simulink model "Simulink_Model"  (R2023a)
settings: Solver=VariableStepAuto  StartTime=0.0  StopTime=0.15  RelTol=1e-3
model workspace (MAT data in the model file):
  y = 0.001
undefined symbols (not defined in the file or in its folder): D1, Delta, x
libraries: spsCurrentMeasurementLib x4, spsDistributedParametersLineLib x3, spsThreePhaseVIMeasurementLib x2, spsThreePhaseParallelRLCLoadLib x1, spsThreePhaseTransformerTwoWindingsLib x1, spsThreePhaseFaultLib x1, spsThreePhaseSourceLib x1, spsVoltageMeasurementLib x1, spspowerguiLib x1
settings Model: Creator=Krish Sanjay Shah  LastModifiedBy=Krish Sanjay Shah

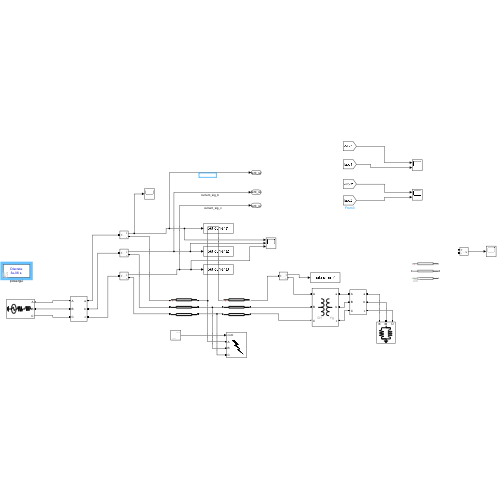
[thumbnail: Simulink's stored preview of the top-level diagram]
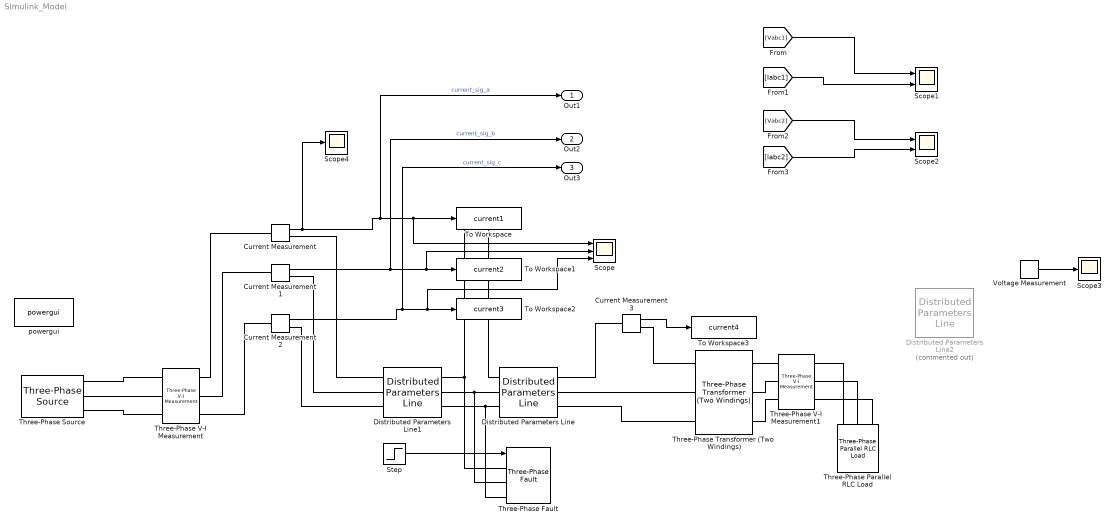
== system Simulink_Model ==
  Current Measurement{,1..3} (4 alike) : spsCurrentMeasurementLib/Current Measurement  PhasorSimulation=off  OutputType=Complex  PSBequivalent=0
  Distributed Parameters Line : spsDistributedParametersLineLib/Distributed Parameters Line  Phases=3  Length=100-x  Frequency=50  Resistance=[0.01273 0.3864]  Inductance="[0.9337e-3  4.1264e-3]"  Capacitance=[12.74e-9 7.751e-9]  x1=[-0.000555 -5.58295531136589e-12 3727.3774424138 -10318.9689781437;-0.000552 -5.5777870589433e-12 3737.10118466611 -10315.4514252007;-0.000549 -5.57261385197143e-12 3746.82160738473 -10311.9247094101;-0.000546 -5.56743569504544e-12 3756.53870193537 -10308.3888339046;-0.000543 -5.56225259276491e-12 3766.25245968668 -10304.8438018251;-0.00054 -5.55706454973381e-12 3775.96287201026 -10301.2896163203;-0.000537 -5.55187157056049e-12 3785.66993028072 -10297.7262805474;-0.000534 -5.54667365985768e-12 3795.3736258756 -10294.1537976716;-0.000531 -5.54147082224252e-12 3805.07395017548 -10290.5721708661;-0.000528 -5.53626306233648e-12 3814.77089456389 -10286.9814033125;-0.000525 -5.53105038476544e-12 3824.46445042739 -10283.3814982002;-0.000522 -5.52583279415963e-12 3834.15460915553 -10279.7724587269;-0.000519 -5.52061029515366e-12 3843.84136214089 -10276.1542880984;-0.000516 -5.51538289238648e-12 3853.52470077909 -10272.5269895286;-0.000513 -5.51015059050141e-12 3863.20461646874 -10268.8905662395;-0.00051 -5.50491339414612e-12 3872.88110061154 -10265.2450214612;-0.000507 -5.49967130797261e-12 3882.55414461219 -10261.5903584319;-0.000504 -5.49442433663725e-12 3892.22373987849 -10257.9265803979;-0.000501 -5.48917248480074e-12 3901.88987782128 -10254.2536906137;-0.000498 -5.48391575712811e-12 3911.55254985446 -10250.5716923416;-0.000495 -5.47865415828872e-12 3921.21174739504 -10246.8805888524;-0.000492 -5.47338769295627e-12 3930.86746186309 -10243.1803834246;-0.000489 -5.46811636580876e-12 3940.51968468179 -10239.471079345;-0.000486 -5.46284018152852e-12 3950.16840727741 -10235.7526799086;-0.000483 -5.45755914480222e-12 3959.81362107934 -10232.0251884181;-0.00048 -5.45227326032079e-12 3969.45531752007 -10228.2886081846;-0.000477 -5.44698253277951e-12 3979.09348803523 -10224.5429425272;-0.000474 -5.44168696687793e-12 3988.72812406358 -10220.7881947731;-0.000471 -5.43638656731993e-12 3998.35921704701 -10217.0243682573;-0.000468 -5.43108133881365e-12 4007.98675843057 -10213.2514663232;-0.000465 -5.42577128607154e-12 4017.61073966246 -10209.4694923222;-0.000462 -5.42045641381034e-12 4027.23115219403 -10205.6784496135;-0.000459 -5.41513672675104e-12 4036.84798747982 -10201.8783415648;-0.000456 -5.40981222961895e-12 4046.46123697754 -10198.0691715514;-0.000453 -5.40448292714363e-12 4056.07089214807 -10194.2509429569;-0.00045 -5.39914882405889e-12 4065.67694445551 -10190.4236591729;-0.000447 -5.39380992510284e-12 4075.27938536714 -10186.5873235991;-0.000444 -5.38846623501783e-12 4084.87820635346 -10182.7419396431;-0.000441 -5.38311775855047e-12 4094.47339888817 -10178.8875107207;-0.000438 -5.37776450045161e-12 4104.06495444821 -10175.0240402555;-0.000435 -5.37240646547637e-12 4113.65286451374 -10171.1515316795;-0.000432 -5.3670436583841e-12 4123.23712056817 -10167.2699884323;-0.000429 -5.3616760839384e-12 4132.81771409814 -10163.3794139619;-0.000426 -5.35630374690707e-12 4142.39463659354 -10159.4798117241;-0.000423 -5.35092665206218e-12 4151.96787954755 -10155.5711851827;-0.00042 -5.34554480418002e-12 4161.53743445659 -10151.6535378097;-0.000417 -5.34015820804108e-12 4171.10329282037 -10147.726873085;-0.000414 -5.33476686843008e-12 4180.66544614187 -10143.7911944964;-0.000411 -5.32937079013596e-12 4190.22388592739 -10139.84650554;-0.000408 -5.32396997795187e-12 4199.77860368648 -10135.8928097196;-0.000405 -5.31856443667515e-12 4209.32959093205 -10131.9301105471;-0.000402 -5.31315417110735e-12 4218.87683918029 -10127.9584115426;-0.000399 -5.30773918605422e-12 4228.42033995072 -10123.9777162338;-0.000396 -5.3023194863257e-12 4237.96008476619 -10119.9880281568;-0.000393 -5.29689507673591e-12 4247.49606515288 -10115.9893508554;-0.00039 -5.29146596210316e-12 4257.02827264032 -10111.9816878814;-0.000387 -5.28603214724994e-12 4266.55669876139 -10107.9650427948;-0.000384 -5.28059363700292e-12 4276.08133505234 -10103.9394191635;-0.000381 -5.27515043619292e-12 4285.60217305276 -10099.9048205631;-0.000378 -5.26970254965496e-12 4295.11920430563 ...(+8296 chars)]  x2=[-0.000555 -8.16324412980977e-12 3109.62540123163 -10027.2164900334;-0.000552 -8.15415122200079e-12 3119.0744476462 -10024.2812841631;-0.000549 -8.14505107115012e-12 3128.52072349819 -10021.3371740814;-0.000546 -8.13594368534112e-12 3137.96422039683 -10018.3841624033;-0.000543 -8.12682907266356e-12 3147.40492995377 -10015.4222517518;-0.00054 -8.1177072412136e-12 3156.84284378318 -10012.4514447581;-0.000537 -8.10857819909387e-12 3166.27795350169 -10009.4717440608;-0.000534 -8.09944195441335e-12 3175.71025072844 -10006.4831523069;-0.000531 -8.09029851528744e-12 3185.13972708505 -10003.4856721509;-0.000528 -8.08114788983794e-12 3194.56637419566 -10000.4793062553;-0.000525 -8.07199008619302e-12 3203.9901836869 -9997.46405729078;-0.000522 -8.06282511248724e-12 3213.41114718795 -9994.43992793549;-0.000519 -8.0536529768615e-12 3222.8292563305 -9991.40692087572;-0.000516 -8.0444736874631e-12 3232.24450274877 -9988.36503880557;-0.000513 -8.03528725244566e-12 3241.65687807955 -9985.31428442703;-0.00051 -8.02609367996917e-12 3251.06637396215 -9982.25466044999;-0.000507 -8.01689297819996e-12 3260.47298203845 -9979.1861695922;-0.000504 -8.00768515531067e-12 3269.87669395291 -9976.10881457929;-0.000501 -7.99847021948029e-12 3279.27750135253 -9973.02259814476;-0.000498 -7.98924817889412e-12 3288.67539588692 -9969.92752302999;-0.000495 -7.98001904174376e-12 3298.07036920826 -9966.82359198423;-0.000492 -7.97078281622713e-12 3307.46241297134 -9963.71080776459;-0.000489 -7.96153951054844e-12 3316.85151883353 -9960.58917313603;-0.000486 -7.95228913291819e-12 3326.23767845482 -9957.4586908714;-0.000483 -7.94303169155316e-12 3335.62088349783 -9954.3193637514;-0.00048 -7.9337671946764e-12 3345.00112562779 -9951.17119456458;-0.000477 -7.92449565051724e-12 3354.37839651257 -9948.01418610733;-0.000474 -7.91521706731126e-12 3363.75268782267 -9944.84834118393;-0.000471 -7.90593145330029e-12 3373.12399123123 -9941.67366260648;-0.000468 -7.89663881673241e-12 3382.49229841408 -9938.49015319493;-0.000465 -7.88733916586194e-12 3391.85760104966 -9935.29781577707;-0.000462 -7.87803250894942e-12 3401.21989081913 -9932.09665318856;-0.000459 -7.86871885426164e-12 3410.57915940629 -9928.88666827286;-0.000456 -7.85939821007157e-12 3419.93539849763 -9925.66786388129;-0.000453 -7.85007058465841e-12 3429.28859978235 -9922.44024287301;-0.00045 -7.84073598630757e-12 3438.63875495233 -9919.20380811499;-0.000447 -7.83139442331062e-12 3447.98585570215 -9915.95856248204;-0.000444 -7.82204590396535e-12 3457.32989372913 -9912.7045088568;-0.000441 -7.81269043657571e-12 3466.67086073329 -9909.44165012973;-0.000438 -7.80332802945184e-12 3476.00874841737 -9906.1699891991;-0.000435 -7.79395869091001e-12 3485.34354848687 -9902.88952897102;-0.000432 -7.7845824292727e-12 3494.67525265002 -9899.60027235941;-0.000429 -7.77519925286848e-12 3504.0038526178 -9896.30222228599;-0.000426 -7.7658091700321e-12 3513.32934010394 -9892.9953816803;-0.000423 -7.75641218910444e-12 3522.65170682494 -9889.6797534797;-0.00042 -7.7470083184325e-12 3531.97094450009 -9886.35534062933;-0.000417 -7.73759756636941e-12 3541.28704485143 -9883.02214608216;-0.000414 -7.7281799412744e-12 3550.59999960381 -9879.68017279894;-0.000411 -7.7187554515128e-12 3559.90980048485 -9876.32942374822;-0.000408 -7.70932410545607e-12 3569.216439225 -9872.96990190637;-0.000405 -7.69988591148172e-12 3578.5199075575 -9869.60161025751;-0.000402 -7.69044087797336e-12 3587.82019721841 -9866.22455179359;-0.000399 -7.68098901332069e-12 3597.11729994662 -9862.83872951433;-0.000396 -7.67153032591946e-12 3606.41120748383 -9859.44414642722;-0.000393 -7.66206482417148e-12 3615.70191157461 -9856.04080554756;-0.00039 -7.65259251648462e-12 3624.98940396635 -9852.62870989842;-0.000387 -7.64311341127279e-12 3634.27367640931 -9849.20786251064;-0.000384 -7.63362751695595e-12 3643.5547206566 -9845.77826642283;-0.000381 -7.62413484196007e-12 3652.83252846418 -9842.33992468137;-0.000378 -7.61463539471716e-12 3662.10709159093 -9838.89284034044 ...(+8275 chars)]  x3=[-0.000555 -5.59033495049164e-14 20.8975033204712 -16.8365307190214;-0.000552 -5.59192310651593e-14 20.9133620932343 -16.8168278114194;-0.000549 -5.59350629543439e-14 20.9292022894038 -16.7971099660291;-0.000546 -5.59508451584073e-14 20.9450238949094 -16.7773772003651;-0.000543 -5.59665776633306e-14 20.9608268956974 -16.7576295319554;-0.00054 -5.59822604551393e-14 20.9766112777306 -16.7378669783411;-0.000537 -5.59978935199029e-14 20.9923770269882 -16.7180895570767;-0.000534 -5.60134768437352e-14 21.008124129466 -16.6982972857296;-0.000531 -5.60290104127939e-14 21.0238525711766 -16.6784901818806;-0.000528 -5.60444942132812e-14 21.0395623381488 -16.6586682631238;-0.000525 -5.60599282314434e-14 21.0552534164283 -16.6388315470661;-0.000522 -5.6075312453571e-14 21.0709257920772 -16.6189800513279;-0.000519 -5.60906468659987e-14 21.0865794511743 -16.5991137935424;-0.000516 -5.61059314551056e-14 21.102214379815 -16.5792327913563;-0.000513 -5.61211662073148e-14 21.1178305641114 -16.5593370624291;-0.00051 -5.61363511090939e-14 21.1334279901922 -16.5394266244334;-0.000507 -5.61514861469547e-14 21.1490066442027 -16.519501495055;-0.000504 -5.61665713074532e-14 21.164566512305 -16.4995616919927;-0.000501 -5.61816065771899e-14 21.1801075806778 -16.4796072329582;-0.000498 -5.61965919428094e-14 21.1956298355166 -16.4596381356765;-0.000495 -5.62115273910008e-14 21.2111332630333 -16.4396544178853;-0.000492 -5.62264129084975e-14 21.226617849457 -16.4196560973355;-0.000489 -5.62412484820772e-14 21.2420835810333 -16.3996431917909;-0.000486 -5.62560340985619e-14 21.2575304440243 -16.3796157190282;-0.000483 -5.62707697448182e-14 21.2729584247093 -16.3595736968371;-0.00048 -5.62854554077569e-14 21.2883675093842 -16.3395171430202;-0.000477 -5.63000910743333e-14 21.3037576843615 -16.3194460753931;-0.000474 -5.63146767315469e-14 21.3191289359708 -16.2993605117842;-0.000471 -5.63292123664419e-14 21.3344812505583 -16.2792604700347;-0.000468 -5.63436979661069e-14 21.3498146144871 -16.2591459679988;-0.000465 -5.63581335176747e-14 21.3651290141371 -16.2390170235434;-0.000462 -5.63725190083227e-14 21.3804244359051 -16.2188736545485;-0.000459 -5.63868544252729e-14 21.3957008662047 -16.1987158789067;-0.000456 -5.64011397557916e-14 21.4109582914664 -16.1785437145233;-0.000453 -5.64153749871897e-14 21.4261966981376 -16.1583571793167;-0.00045 -5.64295601068225e-14 21.4414160726825 -16.1381562912177;-0.000447 -5.64436951020899e-14 21.4566164015823 -16.1179410681702;-0.000444 -5.64577799604362e-14 21.4717976713351 -16.0977115281305;-0.000441 -5.64718146693505e-14 21.4869598684559 -16.0774676890678;-0.000438 -5.64857992163661e-14 21.5021029794768 -16.0572095689641;-0.000435 -5.6499733589061e-14 21.5172269909465 -16.0369371858139;-0.000432 -5.6513617775058e-14 21.532331889431 -16.0166505576244;-0.000429 -5.65274517620241e-14 21.5474176615131 -15.9963497024155;-0.000426 -5.65412355376711e-14 21.5624842937927 -15.9760346382198;-0.000423 -5.65549690897554e-14 21.5775317728866 -15.9557053830824;-0.00042 -5.6568652406078e-14 21.5925600854288 -15.935361955061;-0.000417 -5.65822854744844e-14 21.60756921807 -15.915004372226;-0.000414 -5.65958682828649e-14 21.6225591574782 -15.8946326526603;-0.000411 -5.66094008191544e-14 21.6375298903383 -15.8742468144593;-0.000408 -5.66228830713323e-14 21.6524814033525 -15.8538468757312;-0.000405 -5.66363150274229e-14 21.6674136832398 -15.8334328545963;-0.000402 -5.66496966754951e-14 21.6823267167363 -15.8130047691879;-0.000399 -5.66630280036624e-14 21.6972204905955 -15.7925626376513;-0.000396 -5.66763090000831e-14 21.7120949915876 -15.7721064781447;-0.000393 -5.66895396529601e-14 21.7269502065002 -15.7516363088384;-0.00039 -5.67027199505412e-14 21.7417861221379 -15.7311521479155;-0.000387 -5.67158498811187e-14 21.7566027253226 -15.7106540135713;-0.000384 -5.67289294330297e-14 21.771400002893 -15.6901419240135;-0.000381 -5.67419585946563e-14 21.7861779417055 -15.6696158974622;-0.000378 -5.67549373544249e-14 21.8009365286332 -15.6490759521502 ...(+8276 chars)]  x4=[-0.000555 -6.06778096436729e-15 0.285467066139237 -59.3990605496309;-0.000552 -6.07292661894897e-15 0.34144922674214 -59.398765122266;-0.000549 -6.07806687916656e-15 0.397431084047879 -59.3984169330968;-0.000546 -6.08320174045415e-15 0.453412588329759 -59.3980159824326;-0.000543 -6.08833119825061e-15 0.509393689861408 -59.3975622706294;-0.00054 -6.09345524799964e-15 0.565374338916814 -59.3970557980904;-0.000537 -6.09857388514973e-15 0.621354485770363 -59.3964965652654;-0.000534 -6.10368710515416e-15 0.677334080696882 -59.3958845726511;-0.000531 -6.10879490347106e-15 0.733313073971702 -59.3952198207912;-0.000528 -6.11389727556334e-15 0.789291415870672 -59.3945023102762;-0.000525 -6.11899421689875e-15 0.845269056670229 -59.3937320417433;-0.000522 -6.12408572294987e-15 0.90124594664744 -59.3929090158768;-0.000519 -6.12917178919407e-15 0.957222036080019 -59.3920332334078;-0.000516 -6.13425241111361e-15 1.01319727524641 -59.3911046951141;-0.000513 -6.13932758419553e-15 1.0691716144258 -59.3901234018206;-0.00051 -6.14439730393175e-15 1.12514500389818 -59.3890893543989;-0.000507 -6.14946156581901e-15 1.18111739394439 -59.3880025537675;-0.000504 -6.15452036535892e-15 1.23708873484615 -59.3868630008918;-0.000501 -6.15957369805791e-15 1.29305897688611 -59.385670696784;-0.000498 -6.16462155942729e-15 1.3490280703479 -59.3844256425031;-0.000495 -6.16966394498324e-15 1.40499596551618 -59.3831278391552;-0.000492 -6.17470085024677e-15 1.46096261267666 -59.381777287893;-0.000489 -6.17973227074378e-15 1.51692796211616 -59.3803739899162;-0.000486 -6.18475820200505e-15 1.57289196412266 -59.3789179464713;-0.000483 -6.18977863956622e-15 1.62885456898534 -59.3774091588515;-0.00048 -6.1947935789678e-15 1.6848157269946 -59.3758476283972;-0.000477 -6.19980301575522e-15 1.74077538844215 -59.3742333564953;-0.000474 -6.20480694547877e-15 1.79673350362101 -59.3725663445799;-0.000471 -6.20980536369362e-15 1.85269002282559 -59.3708465941315;-0.000468 -6.21479826595988e-15 1.90864489635171 -59.3690741066778;-0.000465 -6.21978564784251e-15 1.96459807449665 -59.3672488837933;-0.000462 -6.22476750491141e-15 2.02054950755919 -59.3653709270992;-0.000459 -6.22974383274137e-15 2.07649914583968 -59.3634402382636;-0.000456 -6.2347146269121e-15 2.13244693964005 -59.3614568190016;-0.000453 -6.23967988300821e-15 2.18839283926386 -59.3594206710749;-0.00045 -6.24463959661926e-15 2.24433679501637 -59.3573317962921;-0.000447 -6.24959376333969e-15 2.30027875720457 -59.3551901965087;-0.000444 -6.2545423787689e-15 2.35621867613719 -59.3529958736271;-0.000441 -6.25948543851122e-15 2.41215650212481 -59.3507488295963;-0.000438 -6.26442293817589e-15 2.46809218547985 -59.3484490664124;-0.000435 -6.26935487337712e-15 2.52402567651663 -59.3460965861181;-0.000432 -6.27428123973404e-15 2.57995692555144 -59.343691390803;-0.000429 -6.27920203287073e-15 2.63588588290254 -59.3412334826037;-0.000426 -6.28411724841624e-15 2.69181249889023 -59.3387228637033;-0.000423 -6.28902688200455e-15 2.74773672383689 -59.336159536332;-0.00042 -6.2939309292746e-15 2.80365850806703 -59.3335435027667;-0.000417 -6.29882938587031e-15 2.85957780190733 -59.3308747653312;-0.000414 -6.30372224744056e-15 2.91549455568666 -59.3281533263958;-0.000411 -6.30860950963919e-15 2.97140871973617 -59.3253791883781;-0.000408 -6.31349116812501e-15 3.02732024438931 -59.3225523537422;-0.000405 -6.31836721856183e-15 3.08322907998186 -59.319672824999;-0.000402 -6.32323765661842e-15 3.13913517685199 -59.3167406047064;-0.000399 -6.32810247796856e-15 3.19503848534032 -59.3137556954689;-0.000396 -6.33296167829098e-15 3.25093895578993 -59.3107180999379;-0.000393 -6.33781525326943e-15 3.30683653854642 -59.3076278208116;-0.00039 -6.34266319859267e-15 3.36273118395797 -59.304484860835;-0.000387 -6.34750550995442e-15 3.41862284237536 -59.3012892227999;-0.000384 -6.35234218305345e-15 3.47451146415201 -59.2980409095448;-0.000381 -6.3571732135935e-15 3.53039699964407 -59.2947399239551;-0.000378 -6.36199859728334e-15 3.5862793992104 ...(+8297 chars)]  x5=0.000554230735655828  V1=[9.004e-12 1.096e+04 1.096e+04;314.2 314.2 314.2;2.187 0.4167 -1.154]  V2=[2.274e-12 1.05e+04 1.05e+04;314.2 314.2 314.2;0.7585 0.3721 -1.199]  I1=[8.942e-14 26.84 26.84;314.2 314.2 314.2;-2.539 0.9674 -0.6034]  I2=[4.925e-14 59.41 59.41;314.2 314.2 314.2;1.818 0.07624 -1.495]  nHarmo=1  Measurements=None  Decoupling=off  VsMag0=0  VrMag0=0  VsAngle0=0  VrAngle0=0  IsMag0=0  IrMag0=0  IsAngle0=0  IrAngle0=0
      settings: LibrarySourceBlock=sps_lib/Power Grid Elements/Distributed Parameters Line
  Distributed Parameters Line1 : spsDistributedParametersLineLib/Distributed Parameters Line  Phases=3  Length=x  Frequency=50  Resistance=[0.01273 0.3864]  Inductance="[0.9337e-3  4.1264e-3]"  Capacitance=[12.74e-9 7.751e-9]  x1=[-1.2e-05 -1.83954871437303e-12 0 0;-9e-06 -1.83441132626429e-12 5446.91147624279 -9533.87651759339;-6e-06 -1.8292723087134e-12 5455.89452269233 -9528.73869092862;-3e-06 -1.82413166628518e-12 5464.87272286537 -9523.59240022514]  x2=[-1.2e-05 -4.57144213691916e-12 0 0;-9e-06 -4.56545605758146e-12 5434.03223661431 -9531.30405671462;-6e-06 -4.55946592291199e-12 5443.01286429704 -9526.17836958794;-3e-06 -4.55347173823158e-12 5451.98865714558 -9521.04422069681]  x3=[-1.2e-05 -1.5803084134562e-12 0 0;-9e-06 -1.57981970240911e-12 23.5061505546778 -13.1350607237431;-6e-06 -1.57932958806454e-12 23.5185196160898 -13.1129008683509;-3e-06 -1.57883807085782e-12 23.5308677868397 -13.0907293652366]  x4=[-1.2e-05 -5.34003166758131e-13 0 0;-9e-06 -5.32771603259301e-13 16.6074504479067 -57.3277256214439;-6e-06 -5.3153956651846e-13 16.6614731725027 -57.3120480093776;-3e-06 -5.30307057629981e-13 16.7154810973064 -57.2963194890633]  x5=1.13108313399149e-05  V1=[2.274e-12 1.098e+04 1.098e+04;314.2 314.2 314.2;0.9184 0.5165 -1.054]  V2=[9.004e-12 1.096e+04 1.096e+04;314.2 314.2 314.2;2.347 0.5142 -1.057]  I1=[1.903e-12 26.92 26.92;314.2 314.2 314.2;1.493 1.059 -0.5121]  I2=[1.719e-12 59.68 59.68;314.2 314.2 314.2;-0.7165 0.2761 -1.295]  nHarmo=1  Measurements=None  Decoupling=off  VsMag0=0  VrMag0=0  VsAngle0=0  VrAngle0=0  IsMag0=0  IrMag0=0  IsAngle0=0  IrAngle0=0
      settings: LibrarySourceBlock=sps_lib/Power Grid Elements/Distributed Parameters Line
  Distributed Parameters Line2 : spsDistributedParametersLineLib/Distributed Parameters Line  Commented=on  Phases=3  Length=100  Frequency=60  Resistance=[0.01273 0.3864]  Inductance="[0.9337e-3  4.1264e-3]"  Capacitance=[12.74e-9 7.751e-9]  x1=[0 0 0 0; 0.0001244 0 0 0; 0.0002488 0 0 0; 0.0003733 0 0 0; 0.0004977 0 0 0; 0.0006221 0 0 0]  x2=[0 0 0 0; 0.0001244 0 0 0; 0.0002488 0 0 0; 0.0003733 0 0 0; 0.0004977 0 0 0; 0.0006221 0 0 0]  x3=[0 0 0 0; 0.0001244 0 0 0; 0.0002488 0 0 0; 0.0003733 0 0 0; 0.0004977 0 0 0; 0.0006221 0 0 0]  x4=[0 0 0 0; 0.0001244 0 0 0; 0.0002488 0 0 0; 0.0003733 0 0 0; 0.0004977 0 0 0; 0.0006221 0 0 0]  x5=0  V1=ones(3,3)  V2=ones(3,3)  I1=ones(3,3)  I2=ones(3,3)  nHarmo=1  Measurements=None  Decoupling=off  VsMag0=0  VrMag0=0  VsAngle0=0  VrAngle0=0  IsMag0=0  IrMag0=0  IsAngle0=0  IrAngle0=0
      settings: LibrarySourceBlock=sps_lib/Power Grid Elements/Distributed Parameters Line
  Scope : Scope  NumInputPorts=3
  Scope1 : Scope  NumInputPorts=2
  Scope2 : Scope  NumInputPorts=2
  Scope3 : Scope
  Scope4 : Scope
  Step : Step  Time=t  SampleTime=0
  Three-Phase Parallel RLC Load : spsThreePhaseParallelRLCLoadLib/Three-Phase Parallel RLC Load  LConnTagsString=A|B|C  Configuration=Y (grounded)  NominalVoltage=0.4e3  Vabc=[1e3 1e3 1e3]  Vabcp=[1e3 1e3 1e3]  NominalFrequency=50  UnbalancedPower=off  ActivePower=10e3  InductivePower=100  CapacitivePower=0  Pabc=[10e3 9e3 11e3]  QLabc=[100 90 110]  QCabc=[100 90 110]  Pabcp=[10e3 9e3 11e3]  QLabcp=[100 90 110]  QCabcp=[100 90 110]  Measurements=None  LoadType=constant Z
  Three-Phase Transformer (Two Windings) : spsThreePhaseTransformerTwoWindingsLib/Three-Phase Transformer (Two Windings)  Winding1Connection=Delta (D1)  Winding2Connection=Yg  CoreType=Three single-phase transformers  SetSaturation=off  Hysteresis=off  DataFile='hysteresis'  SetInitialFlux=off  Measurements=None  UNITS=pu  NominalPower=[ 100e6 , 50 ]  Winding1=[ 11e3 , 0.002 , 0.08 ]  Winding2=[ 0.4e3 , 0.002 , 0.08 ]  Rm=500  Lm=500  L0=0.5  Saturation=[ 0,0 ; 0.0024,1.2 ; 1.0,1.52 ]  InitialFluxes=[ 0.8 , -0.8 , 0.7 ]  BreakLoop=off  DiscreteSolver=Trapezoidal iterative  DataType=off  TransfoNumber=1
  Three-Phase V-I Measurement : spsThreePhaseVIMeasurementLib/Three-Phase V-I Measurement  VoltageMeasurement=phase-to-ground  SetLabelV=on  LabelV=Vabc1  Vpu=off  VpuLL=off  CurrentMeasurement=yes  SetLabelI=on  LabelI=Iabc1  Ipu=off  Pbase=100e6  Vbase=500e3  OutputType=Complex  PhasorSimulation=off  PSBequivalent=0
  Three-Phase V-I Measurement1 : spsThreePhaseVIMeasurementLib/Three-Phase V-I Measurement  VoltageMeasurement=phase-to-ground  SetLabelV=on  LabelV=Vabc2  Vpu=off  VpuLL=off  CurrentMeasurement=yes  SetLabelI=on  LabelI=Iabc2  Ipu=off  Pbase=100e6  Vbase=500e3  OutputType=Complex  PhasorSimulation=off  PSBequivalent=0
  Three-Phase Fault : spsThreePhaseFaultLib/Three-Phase Fault  InitialStates=0  FaultA=on  FaultB=off  FaultC=off  GroundFault=on  SwitchTimes=0.05  External=on  SwitchStatus=NaN  FaultResistance=y  GroundResistance=0.01  SnubberResistance=1e6  SnubberCapacitance=inf  Measurements=None
  Three-Phase Source : spsThreePhaseSourceLib/Three-Phase Source  InternalConnection=Yg  VoltagePhases=off  Voltage=11e3  PhaseAngle=0  Voltage_phases=[25e3 25e3 25e3]/sqrt(3)  PhaseAngles_phases=[0 -120 +120]  Frequency=50  NonIdealSource=on  SpecifyImpedance=on  Resistance=0.8929  Inductance=16.58e-3  ShortCircuitLevel=100e6  BaseVoltage=11e3  XRratio=7  BusType=swing  Pref=10e3  Qref=0  Prefabc=[10e3, 10e3, 10e3]  Qrefabc=[0, 0, 0]  Qmin=-inf  Qmax=inf
  To Workspace : ToWorkspace  VariableName=current1  SaveFormat=Structure With Time  SampleTime=-1
  To Workspace1 : ToWorkspace  VariableName=current2  SaveFormat=Structure With Time  SampleTime=-1
  To Workspace2 : ToWorkspace  VariableName=current3  SaveFormat=Structure With Time  SampleTime=-1
  To Workspace3 : ToWorkspace  VariableName=current4  SaveFormat=Structure With Time  SampleTime=-1
  Voltage Measurement : spsVoltageMeasurementLib/Voltage Measurement  PhasorSimulation=off  OutputType=Complex  PSBequivalent=0
  powergui : spspowerguiLib/powergui  Priority=1  SimulationMode=Discrete  SampleTime=3e-06  frequency=60  Iterations=50  frequencyindice=50  Pbase=100e6  ErrMax=1e-4  UnitsV=kV  UnitsW=MW  buscounter=0  FunctionMessages=off  echomessages=off  EnableUseOfTLC=off  CurrentSourceSwitches=on  DisableSnubberDevices=off  DisableRonSwitches=off  DisableVfSwitches=off  DisplayEquations=off  AutomaticDiscreteSolvers=off  SolverType=Tustin/Backward Euler (TBE)  Interpol=off  ExternalGateDelay=off  methode=off  Ts=100  x0status=blocks  SPID=on  SwTol=0  HookPort=off  NonlinearTolerance=1e-4  nMaxIteration=100  ContinueOnMaxIteration=off  RestoreLinks=warning  ResistiveCurrentMeasurement=off  Frange=[0:2:500]  Ylog=off  Xlog=on  ShowGrid=off  save=off  variable=ZData  structure=0  ZoomFFT=off  StartTime=0.0  cycles=1  DisplayStyle=1  fundamental=60  FreqAxis=off  MaxFrequency=1000  frequencyindicesteady=1  RmsSteady=1  display=off
  Out1 : Outport
  Out2 : Outport  Port=2
  Out3 : Outport  Port=3
  wires:
  Current Measurement/1 -> Scope4/1, Out1/1, Scope/1, To Workspace/1  "current_sig_a"
  Current Measurement1/1 -> Out2/1, Scope/2, To Workspace1/1  "current_sig_b"
  Current Measurement2/1 -> Out3/1, Scope/3, To Workspace2/1  "current_sig_c"
  Current Measurement3/1 -> To Workspace3/1
  [Iabc2] -> Scope2/2
  [Iabc1] -> Scope1/2
  [Vabc2] -> Scope2/1
  [Vabc1] -> Scope1/1
  Voltage Measurement/1 -> Scope3/1
  Step/1 -> Three-Phase Fault/1
  connections:
  Three-Phase Source/RConn2 -- Three-Phase V-I Measurement/LConn2
  Three-Phase Source/RConn3 -- Three-Phase V-I Measurement/LConn3
  Three-Phase Source/RConn1 -- Three-Phase V-I Measurement/LConn1
  Three-Phase V-I Measurement/RConn3 -- Current Measurement2/LConn1
  Three-Phase V-I Measurement/RConn2 -- Current Measurement1/LConn1
  Three-Phase V-I Measurement/RConn1 -- Current Measurement/LConn1
  Current Measurement/RConn1 -- Distributed Parameters Line1/LConn1
  Current Measurement1/RConn1 -- Distributed Parameters Line1/LConn2
  Current Measurement2/RConn1 -- Distributed Parameters Line1/LConn3
  Distributed Parameters Line/RConn1 -- Current Measurement3/LConn1
  Current Measurement3/RConn1 -- Three-Phase Transformer (Two Windings)/LConn1
  Distributed Parameters Line/RConn3 -- Three-Phase Transformer (Two Windings)/LConn3
  Distributed Parameters Line/RConn2 -- Three-Phase Transformer (Two Windings)/LConn2
  Distributed Parameters Line1/RConn1 -- Three-Phase Fault/LConn1 -- Distributed Parameters Line/LConn1
  Distributed Parameters Line1/RConn2 -- Three-Phase Fault/LConn2 -- Distributed Parameters Line/LConn2
  Distributed Parameters Line1/RConn3 -- Three-Phase Fault/LConn3 -- Distributed Parameters Line/LConn3
  Three-Phase Transformer (Two Windings)/RConn2 -- Three-Phase V-I Measurement1/LConn2
  Three-Phase Transformer (Two Windings)/RConn1 -- Three-Phase V-I Measurement1/LConn1
  Three-Phase Transformer (Two Windings)/RConn3 -- Three-Phase V-I Measurement1/LConn3
  Three-Phase V-I Measurement1/RConn1 -- Three-Phase Parallel RLC Load/LConn1
  Three-Phase V-I Measurement1/RConn2 -- Three-Phase Parallel RLC Load/LConn2
  Three-Phase V-I Measurement1/RConn3 -- Three-Phase Parallel RLC Load/LConn3
